simulink model "model_rlseLQR"  (R2018b)
settings: Solver=VariableStepAuto  StartTime=0.0  StopTime=2  RelTol=1e-3
values from neighbouring files (symbols this model uses):
  A_long = [-0.127582199485 -0.120326518027 0.0123230287539 1.06961513757 -0.67567396364 -4.05064303254 -0.0530588085475 -1.81350154459 -15.9023430516 -51.0981546265 -0.573740058259 -35.7720899763 ... (16 elements, 4x4)]    [env_vars.mat]
  B_long = [3.87534978111  10.1410705056; 5.16747566432  -0.750644051383; -0.972922039439  0.0330465441648; -66.5738506051  0.29117538195]    [env_vars.mat]
  euler_0 = deg2rad([5,5,0])    [Linearize.m]    (also in env_vars.mat = [0.0872664625997 0.0872664625997 0])
  K_lat = [4.17654229775  1.2715659909  0.259712133105; 6.03556648418  1.7716700746  0.955044544874]    [env_vars.mat]
  K_long = lqr(A,B,Q,R,N)    [KlongRLSE.m]    (also in env_vars.mat = [-0.0131288079248  0.201593133818  -1.33138461086  -0.241030)
  Klqr = [-0.0154609901399  0.183342172824  -1.54713654668  -0.245681114058; 0.0136126900225  -0.0100908215941  0.035031817911  0.00688258529699]    [env_vars.mat]
  omega_0 = [0,0,0]    [Linearize.m]    (also in env_vars.mat = [0 0 0])
  P = M^(-1)    [LSE.m]    (also in RLSE.m = P*(I - XU*XU'*P/(alpha+XU'*P*XU)); RLSESIM.m = eye(6)*100; RLSE_ff.m = alpha^2*P*(I - XU*XU'*P/(R/alpha^2+XU'*P*XU)); RLSE_klm.m = (I-K*XU')*P)
  phi_cmd = 0    [Linearize.m]    (also in env_vars.mat)
  r = false    [KlongRLSE.m]
  TAS_cmd = 12    [Linearize.m]    (also in env_vars.mat)
  theta_cmd = 0    [Linearize.m]    (also in env_vars.mat)
  TRIM =     [env_vars.mat]
  u_trim_long = u_trim([2 4])    [Linearize.m]    (also in env_vars.mat = [0.0367583336466 0.362566575663])
  UAV =     [env_vars.mat]    (also in loadDATCOMmodel.m = raw{1,1})
  Vb_0 = [13    1   -0.15]    [Linearize.m]    (also in Trim_UAV.m = [11 0.5 0.5]; env_vars.mat = [13 1 -0.15])
  w_cmd = 0    [Linearize.m]    (also in env_vars.mat)
  x_trim_long = [TAS_cmd w_cmd 0 0]    [Linearize.m]    (also in env_vars.mat = [12 0 0 0])
undefined symbols (not defined in the file or in its folder): F, MIL, Severe
libraries: aerolibasang x8, aerolibwind2 x3, aerolibadyn x2, aerolibactuator x1, aerolibatmos2 x1, shared6dof x1
settings Model: SimulationMode=accelerator  Creator=Carlos  LastModifiedBy=Carlos
settings OptimizationCC: EfficientMapNaN2IntZero=off
settings HardwareCC: TargetBitPerLong=64  TargetBitPerPointer=64  TargetBitPerSizeT=64  TargetBitPerPtrDiffT=64  TargetLongLongMode=on  TargetIntDivRoundTo=Zero  TargetEndianess=LittleEndian  TargetWordSize=64  TargetHWDeviceType=MATLAB Host  ProdEqTarget=off
settings CodeAppCC: MaxIdLength=128
settings GRTTargetCC: TargetLangStandard=C89/C90 (ANSI)  CombineOutputUpdateFcns=off  GRTInterface=on

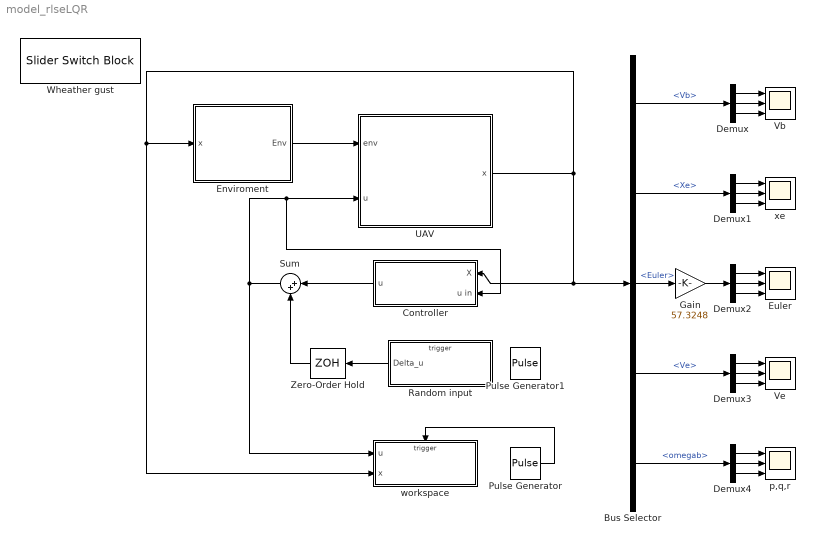
== system model_rlseLQR ==
  Bus Selector : BusSelector  OutputSignals=Vb,Xe,Euler,Ve,omegab
  Controller : Subsystem
  Demux{,1..4} (5 alike) : Demux  Outputs=3
  Enviroment : Subsystem
      mask Display: image('/Volumes/MacintoshHD/Carlos/Downloads/img_7234.png');
  Euler : Scope  NumInputPorts=3
  Gain : Gain  Gain=57.3248
  Pulse Generator : DiscretePulseGenerator  PulseType=Time based  Period=0.02  PulseWidth=5
  Pulse Generator1 : DiscretePulseGenerator  PulseType=Time based  Period=1  PulseWidth=5
  Random input : Subsystem
  Sum : Sum  Inputs=|++
  UAV : Subsystem
      mask Display: image('/Volumes/MacintoshHD/Carlos/Downloads/airplane.gif');
  Vb : Scope  NumInputPorts=3
  Ve : Scope  NumInputPorts=3
  Wheather gust : SliderSwitchBlock  WebBlockId=607
      settings: Values={{'Off', 'On'}, [0 1]}
  Zero-Order Hold : ZeroOrderHold  SampleTime=-1
  p,q,r : Scope  NumInputPorts=3
  workspace : Subsystem  TreatAsAtomicUnit=on
  xe : Scope  NumInputPorts=3
  wires:
  UAV/1("x ") -> Bus Selector/1, Controller/1(X), workspace/2(x), Enviroment/1("x ")
  Enviroment/1(Env) -> UAV/1("env ")
  Demux/1 -> Vb/1
  Bus Selector/1 -> Demux/1  "<Vb>"
  Demux/2 -> Vb/2
  Demux/3 -> Vb/3
  Bus Selector/2 -> Demux1/1  "<Xe>"
  Demux1/1 -> xe/1
  Demux1/2 -> xe/2
  Demux1/3 -> xe/3
  Demux2/1 -> Euler/1
  Demux2/2 -> Euler/2
  Demux2/3 -> Euler/3
  Bus Selector/3 -> Gain/1  "<Euler>"
  Gain/1 -> Demux2/1
  Demux3/3 -> Ve/3
  Bus Selector/4 -> Demux3/1  "<Ve>"
  Demux3/2 -> Ve/2
  Demux3/1 -> Ve/1
  Demux4/1 -> p,q,r/1
  Demux4/3 -> p,q,r/3
  Demux4/2 -> p,q,r/2
  Bus Selector/5 -> Demux4/1  "<omegab>"
  Random input/1(Delta_u) -> Zero-Order Hold/1
  Controller/1(u) -> Sum/1
  Zero-Order Hold/1 -> Sum/2
  Sum/1 -> workspace/1(u), Controller/2(u in), UAV/2(u)
  Pulse Generator/1 -> workspace/Trigger

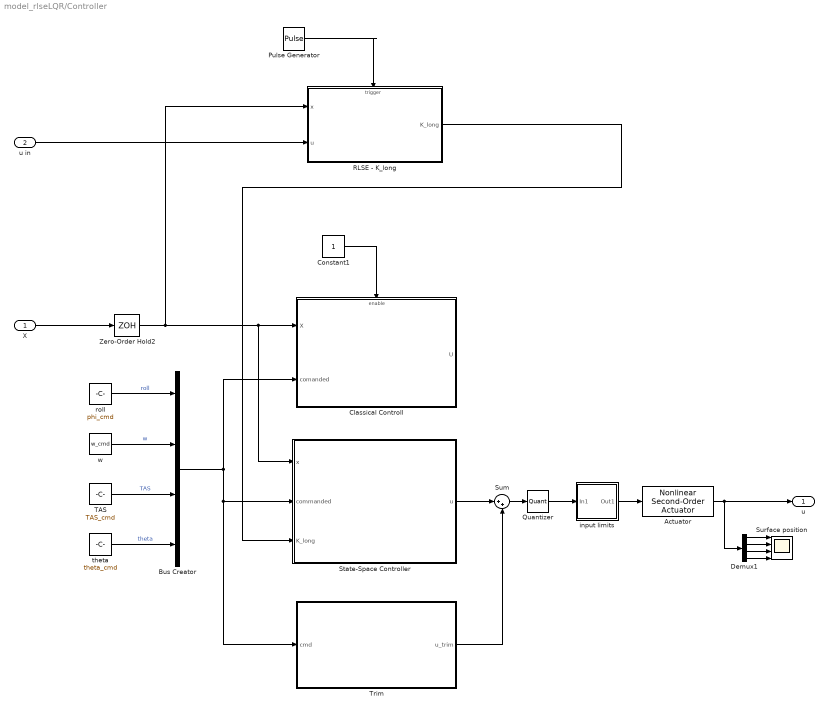
== system model_rlseLQR/Controller ==
  X : Inport
  u in : Inport  Port=2
  Actuator : aerolibactuator/Nonlinear Second-Order Actuator  wn_fin=100  z_fin=0.3  fin_max=1  fin_min=-1  fin_maxrate=2  fin_act_0=0  fin_act_vel=0
      settings: SourceProductName=Aerospace Blockset  SourceProductBaseCode=AE
  Bus Creator : BusCreator  Inputs=4
  Classical Controll : Subsystem  TreatAsAtomicUnit=on
  Constant1 : Constant
  Demux1 : Demux
  Pulse Generator : DiscretePulseGenerator  PulseType=Time based  Period=0.02  PulseWidth=5
  Quantizer : Quantizer  QuantizationInterval=0.004
  RLSE - K_long : Subsystem
  State-Space Controller : Subsystem
  Sum : Sum  Inputs=|++
  Surface position : Scope  NumInputPorts=4
  TAS : Constant  Value=TAS_cmd
  Trim : Subsystem
  Zero-Order Hold2 : ZeroOrderHold  SampleTime=0.01
  input limits : Subsystem
  roll : Constant  Value=phi_cmd
  theta : Constant  Value=theta_cmd
  w : Constant  Value=w_cmd
  u : Outport
  wires:
  Sum/1 -> Quantizer/1
  Constant1/1 -> Classical Controll/Enable
  roll/1 -> Bus Creator/1  "roll"
  Bus Creator/1 -> Classical Controll/2(comanded), Trim/1(cmd), State-Space Controller/2(commanded)
  w/1 -> Bus Creator/2  "w"
  TAS/1 -> Bus Creator/3  "TAS"
  X/1 -> Zero-Order Hold2/1
  Demux1/4 -> Surface position/4
  Demux1/2 -> Surface position/2
  Demux1/1 -> Surface position/1
  Demux1/3 -> Surface position/3
  Zero-Order Hold2/1 -> RLSE - K_long/1(x), State-Space Controller/1(x), Classical Controll/1(X)
  Actuator/1 -> u/1, Demux1/1
  Trim/1(u_trim) -> Sum/2
  theta/1 -> Bus Creator/4  "theta"
  Quantizer/1 -> input limits/1(In1)
  input limits/1(Out1) -> Actuator/1
  Pulse Generator/1 -> RLSE - K_long/Trigger
  RLSE - K_long/1(K_long) -> State-Space Controller/3(K_long)
  u in/1 -> RLSE - K_long/2(u)
  State-Space Controller/1(u) -> Sum/1

== system model_rlseLQR/Enviroment ==
  "x " : Inport
  Bus Creator : BusCreator  Inputs=5
  Bus Selector : BusSelector  OutputSignals=Lhb,Ve,Xe
  Demux : Demux  Outputs=3
  Dot Product : DotProduct  OutDataTypeStr=Inherit: Inherit via internal rule
  ISA Atmosphere Model : aerolibatmos2/ISA Atmosphere Model  custom=off  g=9.80665  gamma=1.4  R=287.0531  L=0.0065  h_trop=11000  h_strat=20000  rho0=1.225  P0=101325  T0=288.15  h0=0
      settings: SourceProductName=Aerospace Blockset
  Scope : Scope  NumInputPorts=3
  Selector : Selector  InputPortWidth=3  IndexOptions=Index vector (dialog)  Indices=[3]  OutputSizes=1
  Wind models : Subsystem
      mask Display: image('/Volumes/MacintoshHD/Carlos/Downloads/f2933471e549912c91ba01f65f304a7c.jpg');
  vt : Sqrt  SaturateOnIntegerOverflow=on
  Env : Outport
  wires:
  Bus Creator/1 -> Env/1
  "x "/1 -> Bus Selector/1
  Bus Selector/3 -> Selector/1  "<Xe>"
  Selector/1 -> ISA Atmosphere Model/1, Wind models/3(altitude)
  ISA Atmosphere Model/4 -> Bus Creator/5  "rho"
  ISA Atmosphere Model/3 -> Bus Creator/4  "P"
  ISA Atmosphere Model/2 -> Bus Creator/3  "a"
  ISA Atmosphere Model/1 -> Bus Creator/2  "T"
  Wind models/1(ug,vg,wg) -> Bus Creator/1, Demux/1  "ug"
  Bus Selector/1 -> Wind models/1(Lhb)  "<Lhb>"
  Dot Product/1 -> vt/1
  Bus Selector/2 -> Dot Product/1, Dot Product/2  "<Ve>"
  vt/1 -> Wind models/2(Airspeed)  "v"
  Demux/1 -> Scope/1
  Demux/2 -> Scope/2
  Demux/3 -> Scope/3

== system model_rlseLQR/Random input ==
  Trigger : TriggerPort  VariantControl=Variant  PortDimensions=1
  random imput vector : MATLAB Function  TreatAsAtomicUnit=on
  Delta_u : Outport
  wires:
  random imput vector/1(y) -> Delta_u/1

== system model_rlseLQR/UAV ==
  "env " : Inport
  u : Inport  Port=2
  6DOF (Euler Angles) : shared6dof/6DOF (Euler Angles)  units=Metric (MKS)  mtype=Fixed  rep=Euler Angles  xme_0=X_0  Vm_0=Vb_0  eul_0=euler_0  pm_0=omega_0  mass_0=UAV.mass  mass_e=0.5  mass_f=2.0  inertia=UAV.Icg  inertia_e=eye(3)  inertia_f=2*eye(3)  k_quat=1.0  vre_flag=on  abi_flag=on  aMode=0  xme_statename=''  Vm_statename=''  eul_statename=''  quat_statename=''  pm_statename=''  mass_statename=''
      settings: SourceProductBaseCode=AE
  Add : Sum  Inputs=3
  "Aero " : Subsystem
  Bus Creator : BusCreator  Inputs=9
  Gravity : Subsystem
  Moto/Propulsion : Subsystem
  Selector : Selector  InputPortWidth=4  IndexOptions=Index vector (dialog)  Indices=[4]  OutputSizes=1
  Sum1 : Sum  Inputs=|++
  "x " : Outport
  wires:
  "env "/1 -> "Aero "/2("Env ")
  6DOF (Euler Angles)/1 -> Bus Creator/1  "Ve"
  6DOF (Euler Angles)/2 -> Bus Creator/2  "Xe"
  6DOF (Euler Angles)/3 -> Bus Creator/3  "Euler"
  6DOF (Euler Angles)/4 -> Bus Creator/4  "Lhb"
  6DOF (Euler Angles)/5 -> [Vb], Bus Creator/5  "Vb"
  Bus Creator/1 -> "Aero "/1("X "), Gravity/1(X), "x "/1
  6DOF (Euler Angles)/6 -> Bus Creator/6  "omegab"
  "Aero "/2("M ") -> Sum1/1
  Moto/Propulsion/2(M) -> Sum1/2
  Selector/1 -> Moto/Propulsion/1(deltap)
  Add/1 -> 6DOF (Euler Angles)/1
  "Aero "/1(F) -> Add/2
  Moto/Propulsion/1(F) -> Add/3
  Sum1/1 -> 6DOF (Euler Angles)/2
  Gravity/1(Fg) -> Add/1
  6DOF (Euler Angles)/7 -> Bus Creator/7  "domegab"
  6DOF (Euler Angles)/8 -> Bus Creator/8  "Abb"
  6DOF (Euler Angles)/9 -> Bus Creator/9  "Abe"
  u/1 -> "Aero "/3(u), Selector/1
  [Vb] -> Moto/Propulsion/2(Vb)

== system model_rlseLQR/workspace ==
  u : Inport
  x : Inport  Port=2
  Trigger : TriggerPort  VariantControl=Variant
  Bus Selector : BusSelector  OutputSignals=Vb,Ve,Euler,omegab,Euler,omegab
  Demux : Demux  Outputs=2
  "Incidence, Sideslip, & Airspeed" : aerolibasang/Incidence, Sideslip, & Airspeed
      settings: SourceProductName=Aerospace Blockset
  Mux : Mux
  Mux1 : Mux
  Selector : Selector  InputPortWidth=4  IndexOptions=Index vector (dialog)  Indices=[2 4]  OutputSizes=1
  Selector1 : Selector  InputPortWidth=4  IndexOptions=Index vector (dialog)  Indices=[1 3]  OutputSizes=1
  Terminator : Terminator
  To Workspace : ToWorkspace  VariableName=u_long  SaveFormat=Timeseries  SampleTime=-1
  To Workspace1 : ToWorkspace  VariableName=x_long  SaveFormat=Timeseries  SampleTime=-1
  To Workspace2 : ToWorkspace  VariableName=u_lat  SaveFormat=Timeseries  SampleTime=-1
  To Workspace3 : ToWorkspace  VariableName=x_lat  SaveFormat=Timeseries  SampleTime=-1
  p,r : Selector  InputPortWidth=3  IndexOptions=Index vector (dialog)  Indices=[1 3]  OutputSizes=1
  phi : Selector  InputPortWidth=3  IndexOptions=Index vector (dialog)  Indices=[1]  OutputSizes=1
  q : Selector  InputPortWidth=3  IndexOptions=Index vector (dialog)  Indices=[2]  OutputSizes=1
  theta : Selector  InputPortWidth=3  IndexOptions=Index vector (dialog)  Indices=[2]  OutputSizes=1
  w : Selector  InputPortWidth=3  IndexOptions=Index vector (dialog)  Indices=[3]  OutputSizes=1
  wires:
  x/1 -> Bus Selector/1
  Bus Selector/2 -> w/1  "<Ve>"
  Bus Selector/3 -> theta/1  "<Euler>"
  Bus Selector/4 -> q/1  "<omegab>"
  Selector/1 -> To Workspace/1
  Mux/1 -> To Workspace1/1
  q/1 -> Mux/4
  theta/1 -> Mux/3
  w/1 -> Mux/2
  Bus Selector/1 -> "Incidence, Sideslip, & Airspeed"/1  "<Vb>"
  "Incidence, Sideslip, & Airspeed"/1 -> Terminator/1
  "Incidence, Sideslip, & Airspeed"/2 -> Mux1/2
  "Incidence, Sideslip, & Airspeed"/3 -> Mux/1
  Selector1/1 -> To Workspace2/1
  u/1 -> Selector1/1, Selector/1
  Bus Selector/6 -> p,r/1  "<omegab>"
  Bus Selector/5 -> phi/1  "<Euler>"
  p,r/1 -> Demux/1
  phi/1 -> Mux1/1
  Demux/2 -> Mux1/4
  Demux/1 -> Mux1/3
  Mux1/1 -> To Workspace3/1

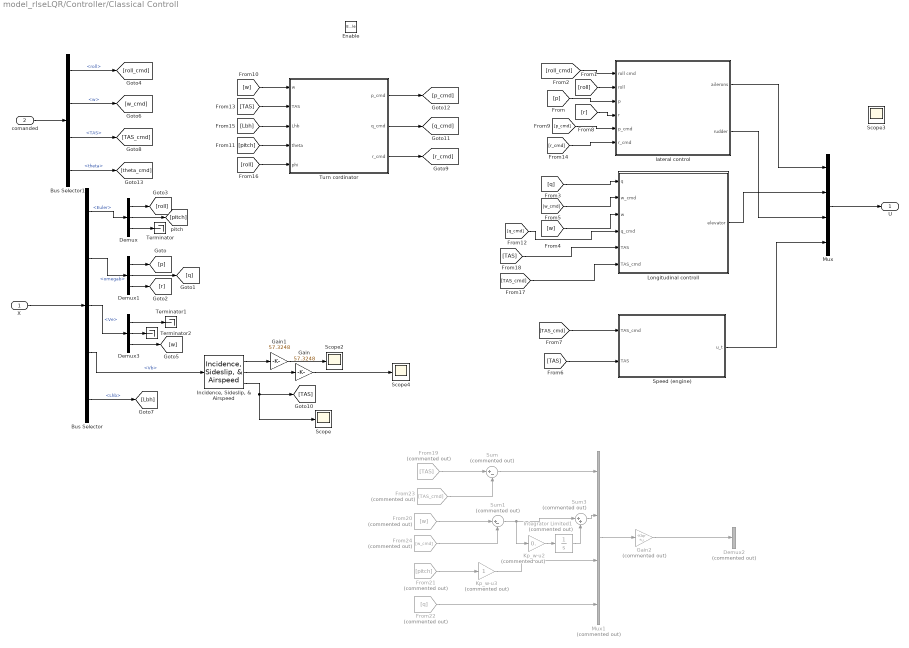
== system model_rlseLQR/Controller/Classical Controll ==
  X : Inport
  comanded : Inport  Port=2
  Enable : EnablePort
  Bus Selector : BusSelector  OutputSignals=Euler,omegab,Ve,Vb,Lhb
  Bus Selector1 : BusSelector  OutputSignals=roll,w,TAS,theta
  Demux : Demux  Outputs=3
  Demux1 : Demux  Outputs=3
  Demux2 : Demux  Commented=on  Outputs=2
  Demux3 : Demux  Outputs=3
  From19 : From  Commented=on  GotoTag=TAS
  From20 : From  Commented=on  GotoTag=w
  From21 : From  Commented=on  GotoTag=pitch
  From22 : From  Commented=on  GotoTag=q
  From23 : From  Commented=on  GotoTag=TAS_cmd
  From24 : From  Commented=on  GotoTag=w_cmd
  Gain : Gain  Gain=57.3248
  Gain1 : Gain  Gain=57.3248
  Gain2 : Gain  Commented=on  Gain=-Klqr  Multiplication=Matrix(K*u)
  "Incidence, Sideslip, & Airspeed" : aerolibasang/Incidence, Sideslip, & Airspeed
      settings: SourceProductName=Aerospace Blockset
  Integrator Limited1 : Integrator  Commented=on  LimitOutput=on  UpperSaturationLimit=2  LowerSaturationLimit=-2
  Kp_w-u2 : Gain  Commented=on  Gain=0.
  Kp_w-u3 : Gain  Commented=on
  Longitudinal controll : Subsystem
  Mux : Mux
  Mux1 : Mux  Commented=on
  Scope{,2..4} (4 alike) : Scope
  Speed (engine) : Subsystem
  Sum : Sum  Commented=on  Inputs=|+-
  Sum1 : Sum  Commented=on  Inputs=|+-
  Sum3 : Sum  Commented=on  Inputs=|++
  Terminator : Terminator
  Terminator1 : Terminator
  Terminator2 : Terminator
  Turn cordinator : Subsystem
  lateral control : Subsystem
  U : Outport
  wires:
  X/1 -> Bus Selector/1
  Bus Selector/1 -> Demux/1  "<Euler>"
  Bus Selector/2 -> Demux1/1  "<omegab>"
  Bus Selector/3 -> Demux3/1  "<Ve>"
  Demux1/1 -> [p]
  Demux1/2 -> [q]
  Demux1/3 -> [r]
  Mux/1 -> U/1
  Demux/1 -> [roll]
  comanded/1 -> Bus Selector1/1
  Bus Selector1/1 -> [roll_cmd]  "<roll>"
  Demux3/3 -> [w]
  Bus Selector1/2 -> [w_cmd]  "<w>"
  [roll_cmd] -> lateral control/1(roll cmd)
  [roll] -> lateral control/2(roll)
  [p] -> lateral control/3(p)
  lateral control/1(ailerons) -> Mux/1
  Bus Selector/4 -> "Incidence, Sideslip, & Airspeed"/1  "<Vb>"
  Bus Selector1/3 -> [TAS_cmd]  "<TAS>"
  "Incidence, Sideslip, & Airspeed"/1 -> Gain1/1
  "Incidence, Sideslip, & Airspeed"/2 -> Gain/1
  Gain/1 -> Scope4/1
  [q] -> Longitudinal controll/1(q)
  [w_cmd] -> Longitudinal controll/2(w_cmd)
  [w] -> Longitudinal controll/3(w)
  lateral control/2(rudder) -> Mux/3
  [r] -> lateral control/4(r)
  [p_cmd] -> lateral control/5(p_cmd)
  [TAS_cmd] -> Speed (engine)/1(TAS_cmd)
  [TAS] -> Speed (engine)/2(TAS)
  [q_cmd] -> Longitudinal controll/4(q_cmd)
  Gain1/1 -> Scope2/1
  Demux/2 -> [pitch]
  [r_cmd] -> lateral control/6(r_cmd)
  "Incidence, Sideslip, & Airspeed"/3 -> [TAS], Scope/1
  Demux/3 -> Terminator/1
  Demux3/1 -> Terminator1/1
  Demux3/2 -> Terminator2/1
  [TAS] -> Turn cordinator/2(TAS)
  Bus Selector/5 -> [Lbh]  "<Lhb>"
  [Lbh] -> Turn cordinator/3(Lhb)
  Turn cordinator/2(q_cmd) -> [q_cmd]
  Turn cordinator/3(r_cmd) -> [r_cmd]
  Turn cordinator/1(p_cmd) -> [p_cmd]
  [w] -> Turn cordinator/1(w)
  [pitch] -> Turn cordinator/4(theta)
  [roll] -> Turn cordinator/5(phi)
  [TAS_cmd] -> Longitudinal controll/6(TAS_cmd)
  [TAS] -> Longitudinal controll/5(TAS)
  From24/1 -> Sum1/2
  From20/1 -> Sum1/1
  From23/1 -> Sum/2
  From19/1 -> Sum/1
  From21/1 -> Kp_w-u3/1
  From22/1 -> Mux1/4
  Mux1/1 -> Gain2/1
  Integrator Limited1/1 -> Sum3/2
  Kp_w-u2/1 -> Integrator Limited1/1
  Sum1/1 -> Kp_w-u2/1, Sum3/1
  Sum3/1 -> Mux1/2
  Kp_w-u3/1 -> Mux1/3
  Sum/1 -> Mux1/1
  Gain2/1 -> Demux2/1
  Speed (engine)/1(u_t) -> Mux/4
  Longitudinal controll/1(elevator) -> Mux/2
  Bus Selector1/4 -> [theta_cmd]  "<theta>"

== system model_rlseLQR/Controller/RLSE - K_long ==
  x : Inport
  u : Inport  Port=2
  Trigger : TriggerPort  VariantControl=Variant  PortDimensions=1
  Bus Selector : BusSelector  OutputSignals=Vb,Ve,Euler,omegab
  Gain : Gain  Gain=50
  "Incidence, Sideslip, & Airspeed" : aerolibasang/Incidence, Sideslip, & Airspeed
      settings: SourceProductName=Aerospace Blockset
  Memory : Memory  InitialCondition=u_trim_long  InheritSampleTime=on
  Memory1 : Memory  InitialCondition=[Vb_0(1) 0 euler_0(2) omega_0(2)]  InheritSampleTime=on
  Mux : Mux
  RLSE & LQR : Subsystem
  Selector : Selector  InputPortWidth=4  IndexOptions=Index vector (dialog)  Indices=[2 4]  OutputSizes=1
  Subtract : Sum  Inputs=-+
  Terminator : Terminator
  Terminator1 : Terminator
  q : Selector  InputPortWidth=3  IndexOptions=Index vector (dialog)  Indices=[2]  OutputSizes=1
  theta : Selector  InputPortWidth=3  IndexOptions=Index vector (dialog)  Indices=[2]  OutputSizes=1
  w : Selector  InputPortWidth=3  IndexOptions=Index vector (dialog)  Indices=[3]  OutputSizes=1
  K_long : Outport
  wires:
  u/1 -> Selector/1
  Subtract/1 -> Gain/1  "∆x"
  Gain/1 -> RLSE & LQR/2(dx)  "dx"
  x/1 -> Bus Selector/1
  w/1 -> Mux/2
  theta/1 -> Mux/3
  q/1 -> Mux/4
  Bus Selector/1 -> "Incidence, Sideslip, & Airspeed"/1  "<Vb>"
  Bus Selector/2 -> w/1  "<Ve>"
  Bus Selector/3 -> theta/1  "<Euler>"
  Bus Selector/4 -> q/1  "<omegab>"
  "Incidence, Sideslip, & Airspeed"/3 -> Mux/1
  "Incidence, Sideslip, & Airspeed"/2 -> Terminator/1
  "Incidence, Sideslip, & Airspeed"/1 -> Terminator1/1
  Memory1/1 -> RLSE & LQR/1(x), Subtract/1
  Selector/1 -> Memory/1
  Mux/1 -> Subtract/2, Memory1/1
  RLSE & LQR/1(K_long) -> K_long/1
  Memory/1 -> RLSE & LQR/3(u)

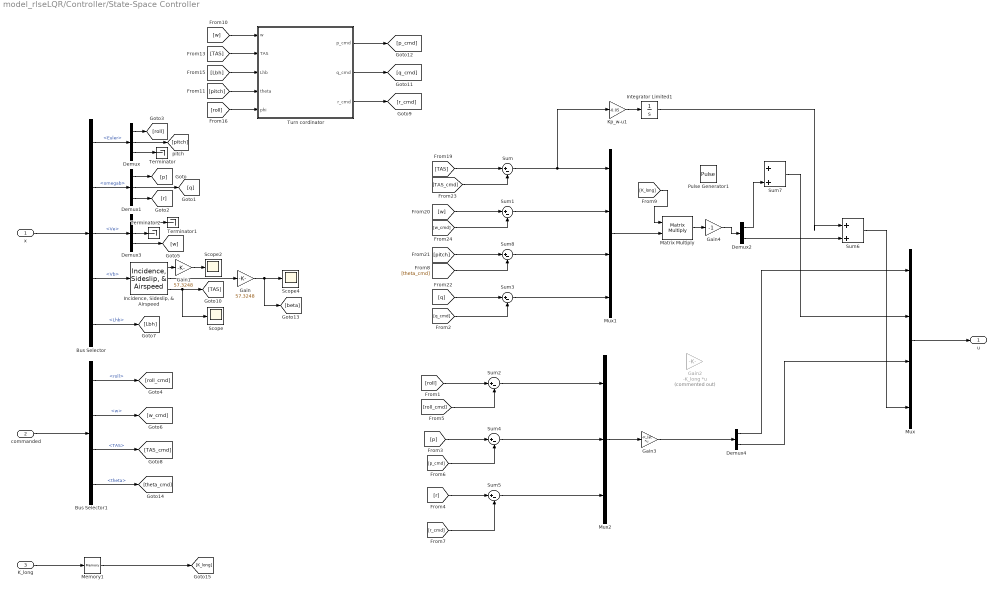
== system model_rlseLQR/Controller/State-Space Controller ==
  x : Inport
  commanded : Inport  Port=2
  K_long : Inport  Port=3
  Bus Selector : BusSelector  OutputSignals=Euler,omegab,Ve,Vb,Lhb
  Bus Selector1 : BusSelector  OutputSignals=roll,w,TAS,theta
  Demux : Demux  Outputs=3
  Demux1 : Demux  Outputs=3
  Demux2 : Demux  Outputs=2
  Demux3 : Demux  Outputs=3
  Demux4 : Demux  Outputs=2
  Gain : Gain  Gain=57.3248
  Gain1 : Gain  Gain=57.3248
  Gain2 : Gain  Commented=on  Gain=-K_long  Multiplication=Matrix(K*u)
  Gain3 : Gain  Gain=-K_lat  Multiplication=Matrix(K*u)
  Gain4 : Gain  Gain=-1
  "Incidence, Sideslip, & Airspeed" : aerolibasang/Incidence, Sideslip, & Airspeed
      settings: SourceProductName=Aerospace Blockset
  Integrator Limited1 : Integrator  LimitOutput=on  UpperSaturationLimit=0.3  LowerSaturationLimit=-0.3
  Kp_w-u1 : Gain  Gain=-0.05
  Matrix Multiply : Product  Multiplication=Matrix(*)
  Memory1 : Memory  InitialCondition=K_long  InheritSampleTime=on
  Mux : Mux
  Mux1 : Mux
  Mux2 : Mux  Inputs=3
  Pulse Generator1 : DiscretePulseGenerator  PulseType=Time based  Amplitude=0.1  Period=1  PulseWidth=10
  Scope : Scope
  Scope2 : Scope
  Scope4 : Scope
  Sum{,1..5,8} (7 alike) : Sum  Inputs=|+-
  Sum6 : Sum  Inputs=|++
  Sum7 : Sum  Inputs=|++
  Terminator : Terminator
  Terminator1 : Terminator
  Terminator2 : Terminator
  Turn cordinator : Subsystem
  u : Outport
  wires:
  Bus Selector1/1 -> [roll_cmd]  "<roll>"
  Bus Selector1/2 -> [w_cmd]  "<w>"
  Bus Selector1/3 -> [TAS_cmd]  "<TAS>"
  commanded/1 -> Bus Selector1/1
  [w_cmd] -> Sum1/2
  [TAS_cmd] -> Sum/2
  [w] -> Sum1/1
  [TAS] -> Sum/1
  Turn cordinator/2(q_cmd) -> [q_cmd]
  Turn cordinator/3(r_cmd) -> [r_cmd]
  Turn cordinator/1(p_cmd) -> [p_cmd]
  [w] -> Turn cordinator/1(w)
  [TAS] -> Turn cordinator/2(TAS)
  [pitch] -> Turn cordinator/4(theta)
  [roll] -> Turn cordinator/5(phi)
  [Lbh] -> Turn cordinator/3(Lhb)
  Bus Selector/1 -> Demux/1  "<Euler>"
  Demux/1 -> [roll]
  Demux3/3 -> [w]
  Bus Selector/3 -> Demux3/1  "<Ve>"
  Bus Selector/2 -> Demux1/1  "<omegab>"
  Gain/1 -> Scope4/1, [beta]
  Demux1/3 -> [r]
  Demux3/1 -> Terminator1/1
  Demux1/1 -> [p]
  Bus Selector/5 -> [Lbh]  "<Lhb>"
  Demux/3 -> Terminator/1
  "Incidence, Sideslip, & Airspeed"/3 -> [TAS], Scope/1
  Demux1/2 -> [q]
  "Incidence, Sideslip, & Airspeed"/2 -> Gain/1
  Demux3/2 -> Terminator2/1
  "Incidence, Sideslip, & Airspeed"/1 -> Gain1/1
  Gain1/1 -> Scope2/1
  Bus Selector/4 -> "Incidence, Sideslip, & Airspeed"/1  "<Vb>"
  Demux/2 -> [pitch]
  x/1 -> Bus Selector/1
  Mux2/1 -> Gain3/1
  Gain3/1 -> Demux4/1
  [roll_cmd] -> Sum2/2
  [roll] -> Sum2/1
  Mux/1 -> u/1
  Demux4/1 -> Mux/1
  Demux4/2 -> Mux/3
  Sum2/1 -> Mux2/1
  Sum1/1 -> Mux1/2
  [q] -> Sum3/1
  Sum3/1 -> Mux1/4
  [q_cmd] -> Sum3/2
  [p] -> Sum4/1
  Sum4/1 -> Mux2/2
  [p_cmd] -> Sum4/2
  [r] -> Sum5/1
  Sum5/1 -> Mux2/3
  [r_cmd] -> Sum5/2
  Integrator Limited1/1 -> Sum6/1
  Kp_w-u1/1 -> Integrator Limited1/1
  Sum/1 -> Kp_w-u1/1, Mux1/1
  Demux2/2 -> Sum6/2
  Sum6/1 -> Mux/4
  Demux2/1 -> Sum7/2
  Sum7/1 -> Mux/2
  Bus Selector1/4 -> [theta_cmd]  "<theta>"
  [theta_cmd] -> Sum8/2
  [pitch] -> Sum8/1
  Sum8/1 -> Mux1/3
  K_long/1 -> Memory1/1
  [K_long] -> Matrix Multiply/1
  Memory1/1 -> [K_long]
  Matrix Multiply/1 -> Gain4/1
  Mux1/1 -> Matrix Multiply/2
  Gain4/1 -> Demux2/1

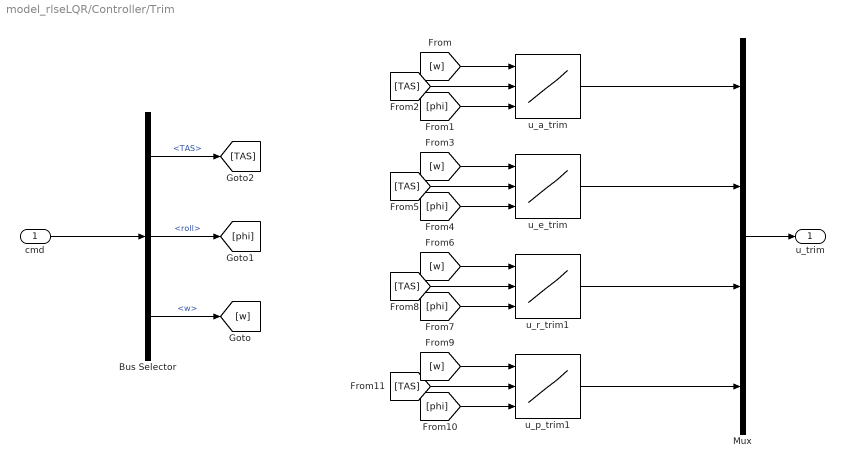
== system model_rlseLQR/Controller/Trim ==
  cmd : Inport
  Bus Selector : BusSelector  OutputSignals=TAS,roll,w
  Mux : Mux
  u_a_trim : Lookup_n-D  NumberOfTableDimensions=3  BreakpointsForDimension1=TRIM.w  BreakpointsForDimension2=TRIM.TAS  BreakpointsForDimension3=TRIM.phi  Table=TRIM.u_a  InternalRulePriority=Speed  RndMeth=Simplest  InputSameDT=on
  u_e_trim : Lookup_n-D  NumberOfTableDimensions=3  BreakpointsForDimension1=TRIM.w  BreakpointsForDimension2=TRIM.TAS  BreakpointsForDimension3=TRIM.phi  Table=TRIM.u_e  InternalRulePriority=Speed  RndMeth=Simplest  InputSameDT=on
  u_p_trim1 : Lookup_n-D  NumberOfTableDimensions=3  BreakpointsForDimension1=TRIM.w  BreakpointsForDimension2=TRIM.TAS  BreakpointsForDimension3=TRIM.phi  Table=TRIM.u_p  InternalRulePriority=Speed  RndMeth=Simplest  InputSameDT=on
  u_r_trim1 : Lookup_n-D  NumberOfTableDimensions=3  BreakpointsForDimension1=TRIM.w  BreakpointsForDimension2=TRIM.TAS  BreakpointsForDimension3=TRIM.phi  Table=TRIM.u_r  InternalRulePriority=Speed  RndMeth=Simplest  InputSameDT=on
  u_trim : Outport
  wires:
  Mux/1 -> u_trim/1
  u_a_trim/1 -> Mux/1
  cmd/1 -> Bus Selector/1
  [w] -> u_a_trim/1
  [phi] -> u_a_trim/3
  [TAS] -> u_a_trim/2
  [TAS] -> u_e_trim/2
  [w] -> u_e_trim/1
  [phi] -> u_e_trim/3
  u_e_trim/1 -> Mux/2
  u_r_trim1/1 -> Mux/3
  [TAS] -> u_r_trim1/2
  [w] -> u_r_trim1/1
  [phi] -> u_r_trim1/3
  u_p_trim1/1 -> Mux/4
  [TAS] -> u_p_trim1/2
  [w] -> u_p_trim1/1
  [phi] -> u_p_trim1/3
  Bus Selector/1 -> [TAS]  "<TAS>"
  Bus Selector/2 -> [phi]  "<roll>"
  Bus Selector/3 -> [w]  "<w>"

== system model_rlseLQR/Controller/input limits ==
  In1 : Inport
  Demux : Demux
  Mux : Mux
  Saturation : Saturate  UpperLimit=1  LowerLimit=-1
  Saturation1 : Saturate  UpperLimit=1  LowerLimit=-1
  Saturation2 : Saturate  UpperLimit=1  LowerLimit=-1
  Saturation3 : Saturate  UpperLimit=1  LowerLimit=0
  Out1 : Outport
  wires:
  In1/1 -> Demux/1
  Demux/1 -> Saturation/1
  Demux/2 -> Saturation1/1
  Demux/3 -> Saturation2/1
  Demux/4 -> Saturation3/1
  Saturation/1 -> Mux/1
  Mux/1 -> Out1/1
  Saturation3/1 -> Mux/4
  Saturation2/1 -> Mux/3
  Saturation1/1 -> Mux/2

== system model_rlseLQR/Enviroment/Wind models ==
  Lhb : Inport
  Airspeed : Inport  Port=2
  altitude : Inport  Port=3
  Discrete Wind Gust Model : aerolibwind2/Discrete Wind Gust Model  units=Metric (MKS)  Gx=off  Gy=off  Gz=off  t_0=20  d_m=[10 10 10]  v_m=[1 1 1]
      settings: SourceProductName=Aerospace Blockset
  Dryden Wind Turbulence Model (Continuous (+q +r)) : aerolibwind2/Dryden Wind Turbulence Model  (Continuous (+q -r))  units=Metric (MKS)  spec=MIL-F-8785C  model=Discrete Dryden (+q +r)  W20=2  Wdeg=90  TurbProb=10^-5 - Severe  L_high=533.4  Wingspan=2  ts=0.1  Seed=[23341 23342 23343 23344]  T_on=on
      settings: SourceProductName=Aerospace Blockset
  Scope : Scope
  Sum : Sum  Inputs=+++  SaturateOnIntegerOverflow=on  InputSameDT=on  OutDataTypeStr=Inherit: Same as first input
  Terminator : Terminator
  Wind Shear Model : aerolibwind2/Wind Shear Model  units=Metric (MKS)  phase=Category C - Terminal Flight Phase  W_20=5  Wdeg=90
      settings: SourceProductName=Aerospace Blockset
  ug,vg,wg : Outport  Unit=m/s
  wires:
  Discrete Wind Gust Model/1 -> Sum/3
  altitude/1 -> Wind Shear Model/1, Dryden Wind Turbulence Model (Continuous (+q +r))/1
  Lhb/1 -> Wind Shear Model/2, Dryden Wind Turbulence Model (Continuous (+q +r))/3
  Dryden Wind Turbulence Model (Continuous (+q +r))/2 -> Terminator/1  "WindAngularRates"
  Airspeed/1 -> Dryden Wind Turbulence Model (Continuous (+q +r))/2, Discrete Wind Gust Model/1
  Sum/1 -> Scope/1, ug,vg,wg/1  "WindVelocity"
  Dryden Wind Turbulence Model (Continuous (+q +r))/1 -> Sum/2
  Wind Shear Model/1 -> Sum/1

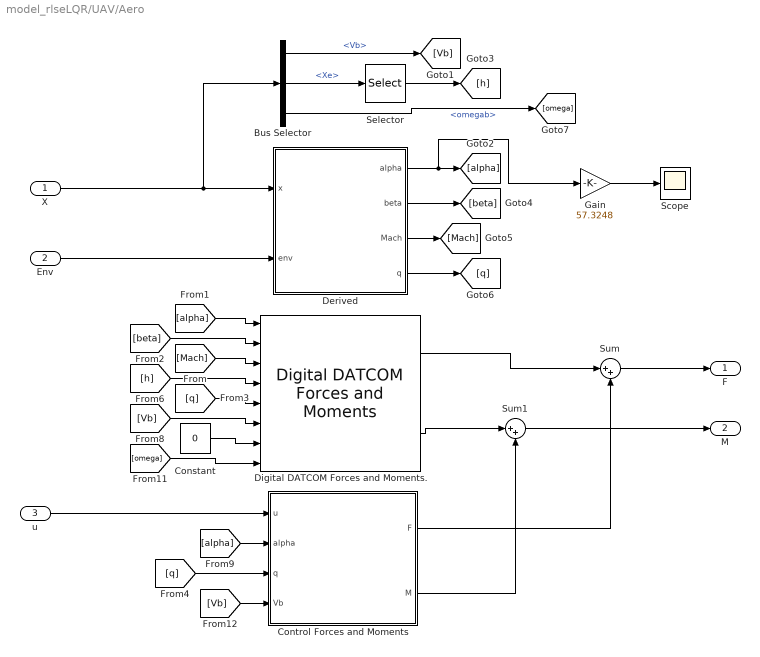
== system model_rlseLQR/UAV/Aero  ==
  "X " : Inport
  "Env " : Inport  Port=2
  u : Inport  Port=3
  Bus Selector : BusSelector  OutputSignals=Vb,Xe,omegab
  Constant : Constant  Value=0
  Control Forces and Moments : Subsystem
  Derived : Subsystem
  Digital DATCOM Forces and Moments. : aerolibadyn/Digital DATCOM Forces and Moments  units=Metric (MKS)  dcase=UAV  fmode=Body  buildno=0  imethod=None - flat  emethod=None - clip  rmethod=Clip to Range  action=None
      settings: SourceProductName=Aerospace Blockset  SourceProductBaseCode=AE
  Gain : Gain  Gain=57.3248
  Scope : Scope
  Selector : Selector  InputPortWidth=3  IndexOptions=Index vector (dialog)  Indices=3  OutputSizes=1
  Sum : Sum  Inputs=|++
  Sum1 : Sum  Inputs=|++
  F : Outport
  "M " : Outport  Port=2
  wires:
  "X "/1 -> Bus Selector/1, Derived/1(x)
  [Mach] -> Digital DATCOM Forces and Moments./3
  Bus Selector/1 -> [Vb]  "<Vb>"
  Digital DATCOM Forces and Moments./2 -> Sum1/1
  Sum1/1 -> "M "/1
  Digital DATCOM Forces and Moments./1 -> Sum/1
  Sum/1 -> F/1
  [q] -> Digital DATCOM Forces and Moments./5
  Control Forces and Moments/1(F) -> Sum/2
  Control Forces and Moments/2(M) -> Sum1/2
  u/1 -> Control Forces and Moments/1(u)
  [q] -> Control Forces and Moments/3(q)
  "Env "/1 -> Derived/2(env)
  Derived/2(beta) -> [beta]
  Derived/4(q) -> [q]
  [alpha] -> Digital DATCOM Forces and Moments./1
  [beta] -> Digital DATCOM Forces and Moments./2
  [h] -> Digital DATCOM Forces and Moments./4
  [Vb] -> Digital DATCOM Forces and Moments./6
  [alpha] -> Control Forces and Moments/2(alpha)
  Bus Selector/2 -> Selector/1  "<Xe>"
  Selector/1 -> [h]
  Bus Selector/3 -> [omega]  "<omegab>"
  Derived/1(alpha) -> Gain/1, [alpha]
  [omega] -> Digital DATCOM Forces and Moments./8
  Derived/3(Mach) -> [Mach]
  Gain/1 -> Scope/1
  [Vb] -> Control Forces and Moments/4(Vb)
  Constant/1 -> Digital DATCOM Forces and Moments./7

== system model_rlseLQR/UAV/Gravity ==
  X : Inport
  Bus Selector : BusSelector  OutputSignals=Lhb
  Constant2 : Constant  Value=[0 0 UAV.mass]
  Gain : Gain  Gain=9.81
  To body Axes : Product  Multiplication=Matrix(*)  SaturateOnIntegerOverflow=on  InputSameDT=on  OutDataTypeStr=Inherit: Same as first input
  Fg : Outport
  wires:
  Bus Selector/1 -> To body Axes/1  "<Lhb>"
  To body Axes/1 -> Fg/1  "Fg"
  X/1 -> Bus Selector/1
  Constant2/1 -> Gain/1
  Gain/1 -> To body Axes/2

== system model_rlseLQR/UAV/Moto//Propulsion ==
  deltap : Inport
  Vb : Inport  Port=2
  Divide : Product  Inputs=*/*
  Divide1 : Product  Inputs=*/*
  Efficiency : Gain  Gain=UAV.eng_eff
  Engine power : Constant  Value=UAV.power
  "Incidence, Sideslip, & Airspeed" : aerolibasang/Incidence, Sideslip, & Airspeed
      settings: SourceProductName=Aerospace Blockset
  Max rpm : Constant  Value=UAV.rpm_max
  Mux : Mux  Inputs=2
  Mux1 : Mux  Inputs=2
  Terminator : Terminator
  Terminator1 : Terminator
  ThrustX1 : Lookup_n-D  NumberOfTableDimensions=1  LookupTableObject=''  BreakpointsForDimension1=(1/6)*(3+([-3:3]))  IndexSearchMethod=Linear search  BeginIndexSearchUsingPreviousIndexResult=on  Table=(0.5*(1+tanh([-3:3])))  ExtrapMethod=Clip  InputSameDT=on
  Ty,Tz : Constant  Value=[0,0]
  Ty,Tz1 : Constant  Value=[0,0]
  rpm2rads : Gain  Gain=0.104719755119660
  F : Outport
  M : Outport  Port=2
  wires:
  Mux/1 -> F/1
  Ty,Tz/1 -> Mux/2
  Ty,Tz1/1 -> Mux1/2
  Mux1/1 -> M/1
  Vb/1 -> "Incidence, Sideslip, & Airspeed"/1
  "Incidence, Sideslip, & Airspeed"/1 -> Terminator/1
  "Incidence, Sideslip, & Airspeed"/2 -> Terminator1/1
  "Incidence, Sideslip, & Airspeed"/3 -> Divide/2
  Engine power/1 -> Divide1/1, Efficiency/1
  ThrustX1/1 -> Divide/3, Divide1/3
  Divide/1 -> Mux/1
  Efficiency/1 -> Divide/1
  deltap/1 -> ThrustX1/1
  Divide1/1 -> Mux1/1
  Max rpm/1 -> rpm2rads/1
  rpm2rads/1 -> Divide1/2

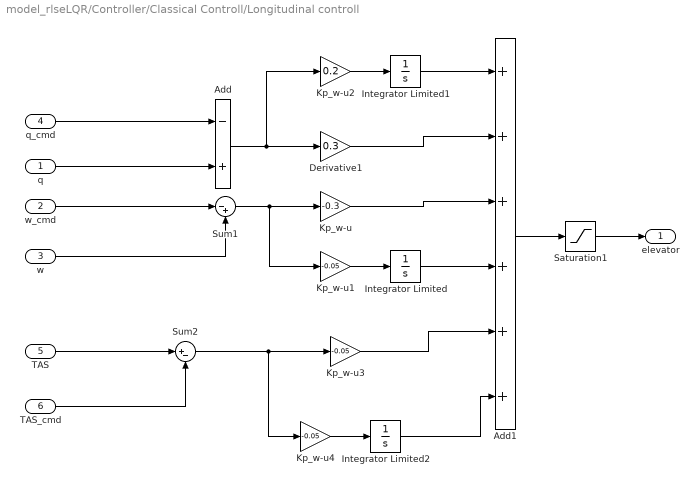
== system model_rlseLQR/Controller/Classical Controll/Longitudinal controll ==
  q : Inport
  w_cmd : Inport  Port=2
  w : Inport  Port=3
  q_cmd : Inport  Port=4
  TAS : Inport  Port=5
  TAS_cmd : Inport  Port=6
  Add : Sum  Inputs=-+
  Add1 : Sum  Inputs=++++++
  Derivative1 : Gain  Gain=0.3
  Integrator Limited : Integrator  LimitOutput=on  UpperSaturationLimit=0.5  LowerSaturationLimit=-0.5
  Integrator Limited1 : Integrator  LimitOutput=on  UpperSaturationLimit=0.25  LowerSaturationLimit=-0.25
  Integrator Limited2 : Integrator  LimitOutput=on  UpperSaturationLimit=0.5  LowerSaturationLimit=-0.5
  Kp_w-u : Gain  Gain=-0.3
  Kp_w-u1 : Gain  Gain=-0.05
  Kp_w-u2 : Gain  Gain=0.2
  Kp_w-u3 : Gain  Gain=-0.05
  Kp_w-u4 : Gain  Gain=-0.05
  Saturation1 : Saturate  UpperLimit=1  LowerLimit=-1
  Sum1 : Sum  Inputs=|-+
  Sum2 : Sum  Inputs=|+-
  elevator : Outport
  wires:
  Saturation1/1 -> elevator/1
  Add1/1 -> Saturation1/1
  w_cmd/1 -> Sum1/1
  Sum1/1 -> Kp_w-u1/1, Kp_w-u/1
  w/1 -> Sum1/2
  Add/1 -> Kp_w-u2/1, Derivative1/1
  q/1 -> Add/2
  Kp_w-u1/1 -> Integrator Limited/1
  q_cmd/1 -> Add/1
  Kp_w-u2/1 -> Integrator Limited1/1
  Integrator Limited/1 -> Add1/4
  Kp_w-u/1 -> Add1/3
  Derivative1/1 -> Add1/2
  Integrator Limited1/1 -> Add1/1
  TAS/1 -> Sum2/1
  TAS_cmd/1 -> Sum2/2
  Kp_w-u3/1 -> Add1/5
  Integrator Limited2/1 -> Add1/6
  Sum2/1 -> Kp_w-u4/1, Kp_w-u3/1
  Kp_w-u4/1 -> Integrator Limited2/1

== system model_rlseLQR/Controller/Classical Controll/Speed (engine) ==
  TAS_cmd : Inport
  TAS : Inport  Port=2
  Add2 : Sum
  Integrator Limited1 : Integrator  LimitOutput=on  UpperSaturationLimit=0.3  LowerSaturationLimit=-0.3
  Kp_w-u1 : Gain  Gain=-0.07
  Saturation2 : Saturate
  Sum2 : Sum  Inputs=|-+
  TAS_prop : Gain  Gain=-0.15
  u_t : Outport
  wires:
  Saturation2/1 -> u_t/1
  TAS_cmd/1 -> Sum2/1
  Add2/1 -> Saturation2/1
  TAS_prop/1 -> Add2/1
  Integrator Limited1/1 -> Add2/2
  TAS/1 -> Sum2/2
  Sum2/1 -> Kp_w-u1/1, TAS_prop/1
  Kp_w-u1/1 -> Integrator Limited1/1

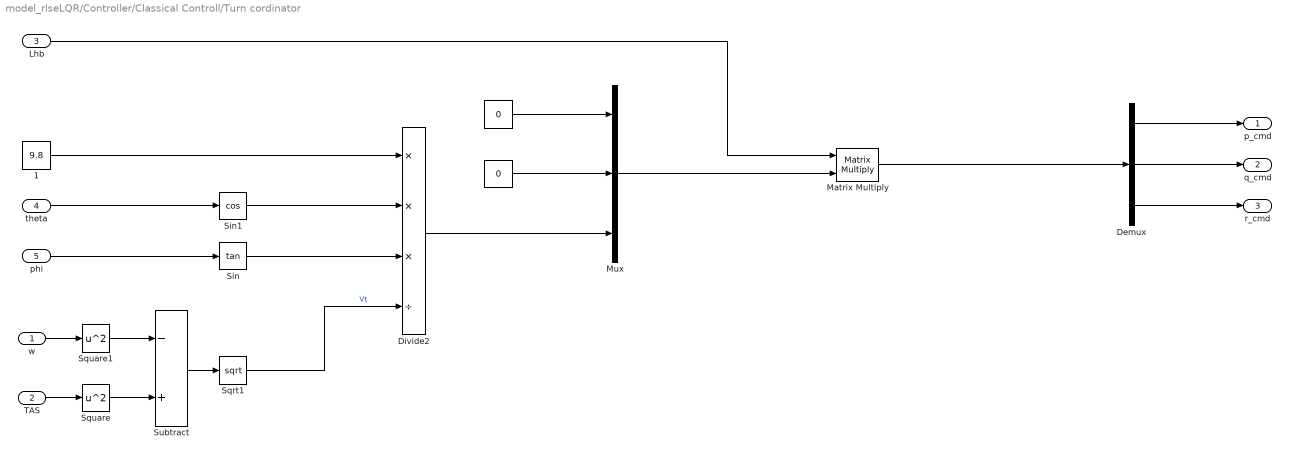
== system model_rlseLQR/Controller/Classical Controll/Turn cordinator ==
  w : Inport
  TAS : Inport  Port=2
  Lhb : Inport  Port=3
  theta : Inport  Port=4
  phi : Inport  Port=5
  " " : Constant  Value=0
  "  " : Constant  Value=0
  " 1" : Constant  Value=9.8
  Demux : Demux  Outputs=3
  Divide2 : Product  Inputs=***/
  Matrix Multiply : Product  Multiplication=Matrix(*)
  Mux : Mux  Inputs=3
  Sin : Trigonometry  Operator=tan  OutputSignalType=real
  Sin1 : Trigonometry  Operator=cos
  Sqrt1 : Sqrt  SaturateOnIntegerOverflow=on
  Square : Math  Operator=square  SaturateOnIntegerOverflow=on
  Square1 : Math  Operator=square  SaturateOnIntegerOverflow=on
  Subtract : Sum  Inputs=-+
  p_cmd : Outport
  q_cmd : Outport  Port=2
  r_cmd : Outport  Port=3
  wires:
  Demux/1 -> p_cmd/1
  Demux/2 -> q_cmd/1
  Demux/3 -> r_cmd/1
  w/1 -> Square1/1
  Square1/1 -> Subtract/1
  Square/1 -> Subtract/2
  Subtract/1 -> Sqrt1/1
  " "/1 -> Mux/1
  theta/1 -> Sin1/1
  phi/1 -> Sin/1
  Sin/1 -> Divide2/3
  Sin1/1 -> Divide2/2
  " 1"/1 -> Divide2/1
  "  "/1 -> Mux/2
  Divide2/1 -> Mux/3
  Lhb/1 -> Matrix Multiply/1
  Mux/1 -> Matrix Multiply/2
  Matrix Multiply/1 -> Demux/1
  TAS/1 -> Square/1
  Sqrt1/1 -> Divide2/4  "Vt"

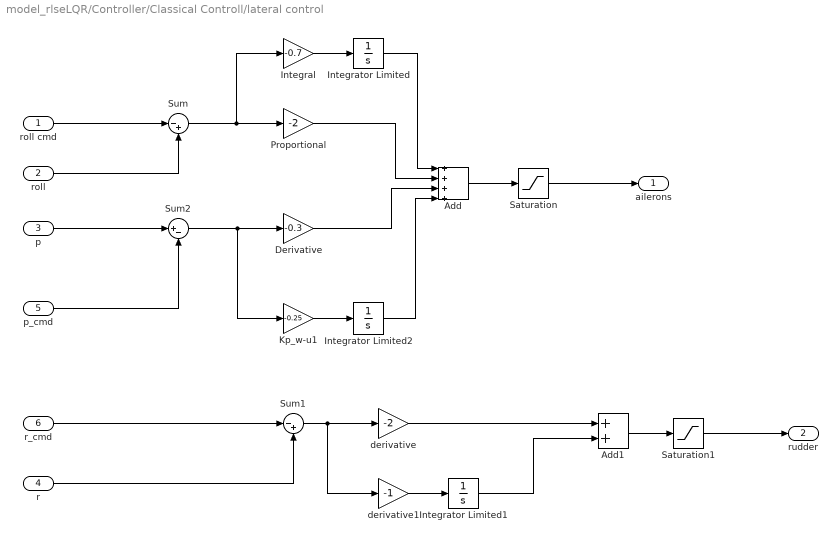
== system model_rlseLQR/Controller/Classical Controll/lateral control ==
  roll cmd : Inport
  roll : Inport  Port=2
  p : Inport  Port=3
  r : Inport  Port=4
  p_cmd : Inport  Port=5
  r_cmd : Inport  Port=6
  Add : Sum  Inputs=++++
  Add1 : Sum
  Derivative : Gain  Gain=-0.3
  Integral : Gain  Gain=-0.7
  Integrator Limited : Integrator  LimitOutput=on  UpperSaturationLimit=0.5  LowerSaturationLimit=-0.5
  Integrator Limited1 : Integrator  LimitOutput=on  UpperSaturationLimit=0.1  LowerSaturationLimit=-0.1
  Integrator Limited2 : Integrator  LimitOutput=on  UpperSaturationLimit=0.25  LowerSaturationLimit=-0.25
  Kp_w-u1 : Gain  Gain=-0.25
  Proportional : Gain  Gain=-2
  Saturation : Saturate  UpperLimit=1  LowerLimit=-1
  Saturation1 : Saturate  UpperLimit=1  LowerLimit=-1
  Sum : Sum  Inputs=|-+
  Sum1 : Sum  Inputs=|-+
  Sum2 : Sum  Inputs=|+-
  derivative : Gain  Gain=-2
  derivative1 : Gain  Gain=-1
  ailerons : Outport
  rudder : Outport  Port=2
  wires:
  roll cmd/1 -> Sum/1
  Saturation/1 -> ailerons/1
  roll/1 -> Sum/2
  Derivative/1 -> Add/3
  Proportional/1 -> Add/2
  Add/1 -> Saturation/1
  Sum/1 -> Proportional/1, Integral/1
  Integral/1 -> Integrator Limited/1
  Integrator Limited/1 -> Add/1
  Add1/1 -> Saturation1/1
  r/1 -> Sum1/2
  Sum1/1 -> derivative1/1, derivative/1
  Integrator Limited1/1 -> Add1/2
  derivative1/1 -> Integrator Limited1/1
  Saturation1/1 -> rudder/1
  r_cmd/1 -> Sum1/1
  p/1 -> Sum2/1
  p_cmd/1 -> Sum2/2
  derivative/1 -> Add1/1
  Sum2/1 -> Kp_w-u1/1, Derivative/1
  Integrator Limited2/1 -> Add/4
  Kp_w-u1/1 -> Integrator Limited2/1

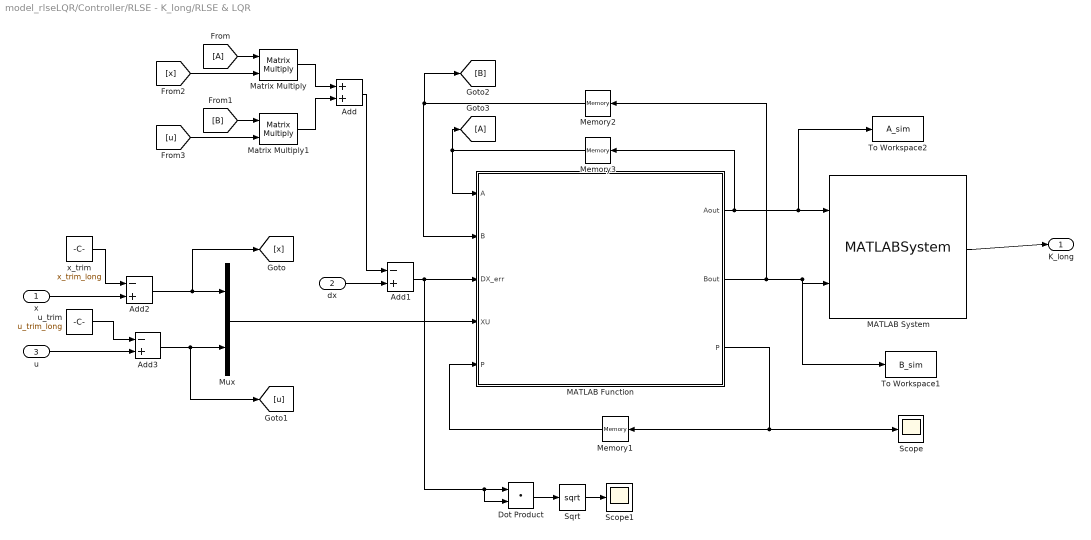
== system model_rlseLQR/Controller/RLSE - K_long/RLSE & LQR ==
  x : Inport
  dx : Inport  Port=2
  u : Inport  Port=3
  Add : Sum
  Add1 : Sum  Inputs=-+
  Add2 : Sum  Inputs=-+
  Add3 : Sum  Inputs=-+
  Dot Product : DotProduct  InputSameDT=on  OutDataTypeStr=Inherit: Inherit via internal rule
  MATLAB Function : MATLAB Function  TreatAsAtomicUnit=on
  MATLAB System : MATLABSystem  System=KlongRLSE  SimulateUsing=Interpreted execution
      mask Type: KlongRLSE
      mask Display:
      | disp('KlongRLSE');
      | port_label('input',1,'A');
      | port_label('input',2,'B');
      | port_label('output',1,'K_long');
  Matrix Multiply : Product  Multiplication=Matrix(*)
  Matrix Multiply1 : Product  Multiplication=Matrix(*)
  Memory1 : Memory  InitialCondition=eye(6)*P  InheritSampleTime=on
  Memory2 : Memory  InitialCondition=B_long  InheritSampleTime=on
  Memory3 : Memory  InitialCondition=A_long  InheritSampleTime=on
  Mux : Mux  Inputs=2
  Scope : Scope
  Scope1 : Scope
  Sqrt : Sqrt  SaturateOnIntegerOverflow=on
  To Workspace1 : ToWorkspace  VariableName=B_sim  SaveFormat=Timeseries  SampleTime=-1
  To Workspace2 : ToWorkspace  VariableName=A_sim  SaveFormat=Timeseries  SampleTime=-1
  u_trim : Constant  Value=u_trim_long
  x_trim : Constant  Value=x_trim_long
  K_long : Outport
  wires:
  Mux/1 -> MATLAB Function/4(XU)
  MATLAB Function/1(Aout) -> Memory3/1, MATLAB System/1, To Workspace2/1
  MATLAB Function/2(Bout) -> Memory2/1, MATLAB System/2, To Workspace1/1
  Memory2/1 -> [B], MATLAB Function/2(B)
  Memory3/1 -> MATLAB Function/1(A), [A]
  Matrix Multiply/1 -> Add/1
  Matrix Multiply1/1 -> Add/2
  [A] -> Matrix Multiply/1
  [B] -> Matrix Multiply1/1
  [u] -> Matrix Multiply1/2
  [x] -> Matrix Multiply/2
  dx/1 -> Add1/2
  Add1/1 -> Dot Product/1, Dot Product/2, MATLAB Function/3(DX_err)
  Add/1 -> Add1/1
  Memory1/1 -> MATLAB Function/5("P ")
  MATLAB Function/3(P) -> Scope/1, Memory1/1
  x/1 -> Add2/2
  Add2/1 -> [x], Mux/1
  u/1 -> Add3/2
  Add3/1 -> [u], Mux/2
  x_trim/1 -> Add2/1
  u_trim/1 -> Add3/1
  MATLAB System/1 -> K_long/1
  Dot Product/1 -> Sqrt/1
  Sqrt/1 -> Scope1/1

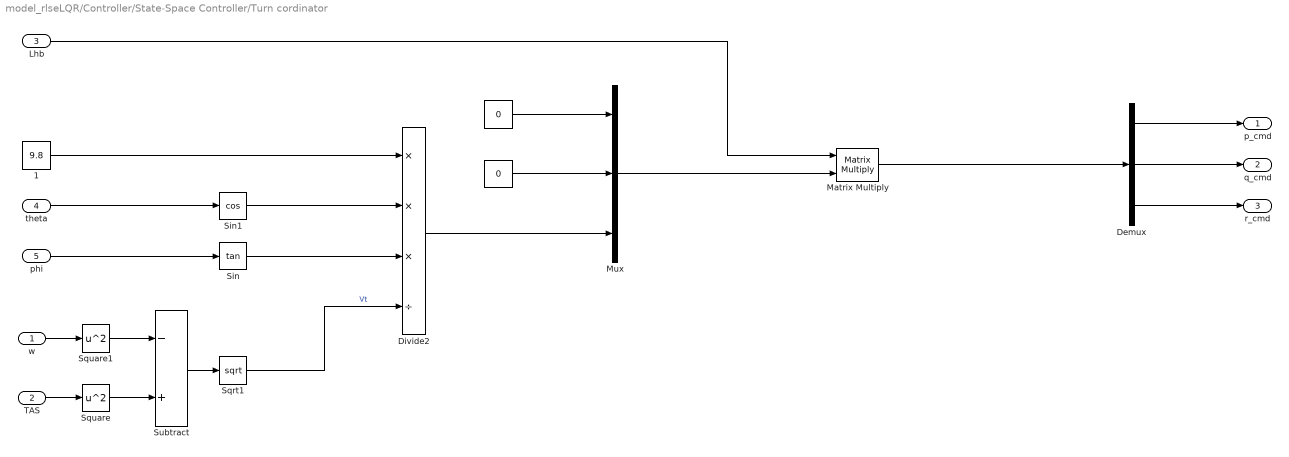
== system model_rlseLQR/Controller/State-Space Controller/Turn cordinator ==
  w : Inport
  TAS : Inport  Port=2
  Lhb : Inport  Port=3
  theta : Inport  Port=4
  phi : Inport  Port=5
  " " : Constant  Value=0
  "  " : Constant  Value=0
  " 1" : Constant  Value=9.8
  Demux : Demux  Outputs=3
  Divide2 : Product  Inputs=***/
  Matrix Multiply : Product  Multiplication=Matrix(*)
  Mux : Mux  Inputs=3
  Sin : Trigonometry  Operator=tan  OutputSignalType=real
  Sin1 : Trigonometry  Operator=cos
  Sqrt1 : Sqrt  SaturateOnIntegerOverflow=on
  Square : Math  Operator=square  SaturateOnIntegerOverflow=on
  Square1 : Math  Operator=square  SaturateOnIntegerOverflow=on
  Subtract : Sum  Inputs=-+
  p_cmd : Outport
  q_cmd : Outport  Port=2
  r_cmd : Outport  Port=3
  wires:
  Demux/1 -> p_cmd/1
  Demux/2 -> q_cmd/1
  Demux/3 -> r_cmd/1
  w/1 -> Square1/1
  Square1/1 -> Subtract/1
  Square/1 -> Subtract/2
  Subtract/1 -> Sqrt1/1
  " "/1 -> Mux/1
  theta/1 -> Sin1/1
  phi/1 -> Sin/1
  Sin/1 -> Divide2/3
  Sin1/1 -> Divide2/2
  " 1"/1 -> Divide2/1
  "  "/1 -> Mux/2
  Divide2/1 -> Mux/3
  Lhb/1 -> Matrix Multiply/1
  Mux/1 -> Matrix Multiply/2
  Matrix Multiply/1 -> Demux/1
  TAS/1 -> Square/1
  Sqrt1/1 -> Divide2/4  "Vt"

== system model_rlseLQR/UAV/Aero /Control Forces and Moments ==
  u : Inport
  alpha : Inport  Port=2
  q : Inport  Port=3
  Vb : Inport  Port=4
  Aero Coefficients : Subsystem
  "Aerodynamic Forces and Moments " : aerolibadyn/Aerodynamic Forces and Moments   inputAxes=Stability  outputForceAxes=Body  outputMomentAxes=Body  S=UAV.sref  b=UAV.blref  cbar=UAV.blref
      settings: SourceProductName=Aerospace Blockset
  F : Outport
  M : Outport  Port=2
  wires:
  "Aerodynamic Forces and Moments "/2 -> M/1
  "Aerodynamic Forces and Moments "/1 -> F/1
  Aero Coefficients/1("Coeff ") -> "Aerodynamic Forces and Moments "/1
  Aero Coefficients/4("Cp ") -> "Aerodynamic Forces and Moments "/4
  alpha/1 -> Aero Coefficients/2(alpha)
  u/1 -> Aero Coefficients/1(u)
  Aero Coefficients/2(qout) -> "Aerodynamic Forces and Moments "/2
  q/1 -> Aero Coefficients/3(q)
  Vb/1 -> "Aerodynamic Forces and Moments "/5
  Aero Coefficients/3("Cg ") -> "Aerodynamic Forces and Moments "/3

== system model_rlseLQR/UAV/Aero /Derived ==
  x : Inport
  env : Inport  Port=2
  Bus Selector : BusSelector  OutputSignals=Vb
  Bus Selector1 : BusSelector  OutputSignals=ug,a,rho
  Dynamic Pressure : aerolibasang/Dynamic Pressure
  Gain : Gain
  "Incidence, Sideslip, & Airspeed" : aerolibasang/Incidence, Sideslip, & Airspeed
      settings: SourceProductName=Aerospace Blockset
  Mach Number : aerolibasang/Mach Number
      settings: SourceProductName=Aerospace Blockset  SourceProductBaseCode=AE
  Sum : Sum  Inputs=|+-
  Terminator : Terminator
  alpha : Outport
  beta : Outport  Port=2
  Mach : Outport  Port=3
  q : Outport  Port=4
  wires:
  x/1 -> Bus Selector/1
  env/1 -> Bus Selector1/1
  Dynamic Pressure/1 -> q/1
  Bus Selector/1 -> Sum/1  "<Vb>"
  Mach Number/1 -> Mach/1  "Mach"
  Bus Selector1/2 -> Mach Number/2  "<a>"
  Bus Selector1/3 -> Dynamic Pressure/2  "<rho>"
  Sum/1 -> Mach Number/1, Dynamic Pressure/1, "Incidence, Sideslip, & Airspeed"/1
  "Incidence, Sideslip, & Airspeed"/1 -> alpha/1
  "Incidence, Sideslip, & Airspeed"/2 -> beta/1
  "Incidence, Sideslip, & Airspeed"/3 -> Terminator/1
  Gain/1 -> Sum/2
  Bus Selector1/1 -> Gain/1  "<ug>"

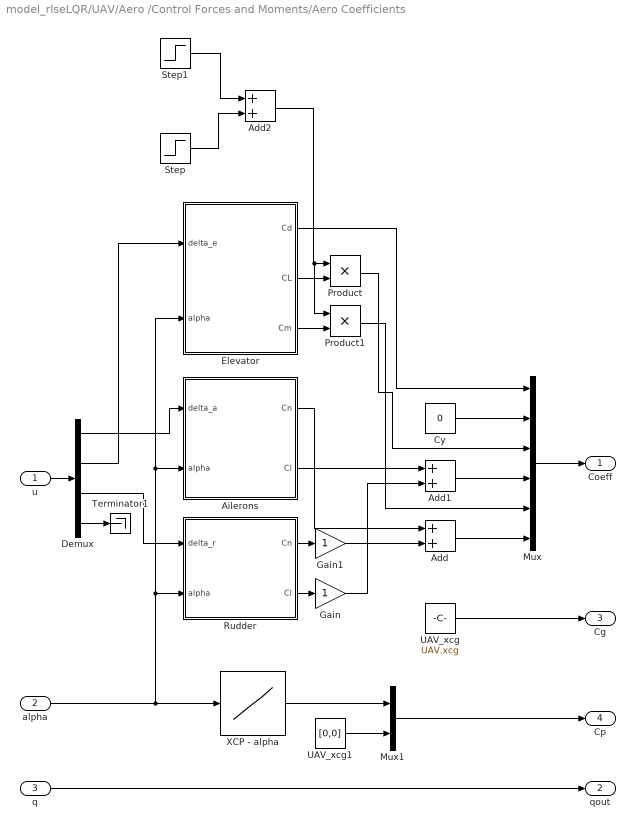
== system model_rlseLQR/UAV/Aero /Control Forces and Moments/Aero Coefficients ==
  u : Inport
  alpha : Inport  Port=2
  q : Inport  Port=3
  Add : Sum
  Add1 : Sum
  Add2 : Sum
  Ailerons : Subsystem
  Cy : Constant  Value=0
  Demux : Demux
  Elevator : Subsystem
  Gain : Gain
  Gain1 : Gain
  Mux : Mux  Inputs=6
  Mux1 : Mux  Inputs=2
  Product : Product
  Product1 : Product
  Rudder : Subsystem
  Step : Step  Time=10  Before=2  After=2  SampleTime=0
  Step1 : Step  Time=10  After=0  SampleTime=0
  Terminator1 : Terminator
  UAV_xcg : Constant  Value=UAV.xcg
  UAV_xcg1 : Constant  Value=[0,0]
  XCP - alpha : Lookup_n-D  NumberOfTableDimensions=1  BreakpointsForDimension1=UAV.alpha  Table=UAV.xcp  InternalRulePriority=Speed  RndMeth=Simplest  InputSameDT=on
  "Coeff " : Outport
  qout : Outport  Port=2
  "Cg " : Outport  Port=3
  "Cp " : Outport  Port=4
  wires:
  q/1 -> qout/1
  alpha/1 -> Rudder/2(alpha), Elevator/2(alpha), Ailerons/2(alpha), XCP - alpha/1
  u/1 -> Demux/1
  Elevator/3(Cm) -> Product1/2
  Elevator/2(CL) -> Product/2
  Demux/1 -> Ailerons/1(delta_a)
  Elevator/1(Cd) -> Mux/1
  Demux/4 -> Terminator1/1
  Cy/1 -> Mux/2
  Demux/3 -> Rudder/1(delta_r)
  Add/1 -> Mux/6
  Ailerons/1(Cn) -> Add/1
  Rudder/1(Cn) -> Gain1/1
  Add1/1 -> Mux/4
  Ailerons/2(Cl) -> Add1/1
  Rudder/2(Cl) -> Gain/1
  UAV_xcg/1 -> "Cg "/1
  Mux1/1 -> "Cp "/1
  XCP - alpha/1 -> Mux1/1
  UAV_xcg1/1 -> Mux1/2
  Mux/1 -> "Coeff "/1
  Demux/2 -> Elevator/1(delta_e)
  Gain/1 -> Add1/2
  Gain1/1 -> Add/2
  Product/1 -> Mux/3
  Product1/1 -> Mux/5
  Step/1 -> Add2/2
  Add2/1 -> Product1/1, Product/1
  Step1/1 -> Add2/1

== system model_rlseLQR/UAV/Aero /Control Forces and Moments/Aero Coefficients/Ailerons ==
  delta_a : Inport
  alpha : Inport  Port=2
  angle(right) - Cl : Lookup_n-D  NumberOfTableDimensions=1  BreakpointsForDimension1=UAV.deltar  Table=UAV.clroll  InternalRulePriority=Speed  RndMeth=Simplest  InputSameDT=on
  angle(right) - Cn : Lookup_n-D  BreakpointsForDimension1=UAV.alpha  BreakpointsForDimension2=UAV.deltar  Table=UAV.cn_asy  InternalRulePriority=Speed  RndMeth=Simplest  InputSameDT=on
  delta_a - aileron (right) angle : Lookup_n-D  NumberOfTableDimensions=1  BreakpointsForDimension1=linspace(-1,1,UAV.ndelta)  Table=UAV.deltal  InternalRulePriority=Speed  RndMeth=Simplest  InputSameDT=on
  Cn : Outport
  Cl : Outport  Port=2
  wires:
  delta_a/1 -> delta_a - aileron (right) angle/1
  angle(right) - Cl/1 -> Cl/1
  delta_a - aileron (right) angle/1 -> angle(right) - Cn/2, angle(right) - Cl/1  "Surface angle"
  alpha/1 -> angle(right) - Cn/1
  angle(right) - Cn/1 -> Cn/1

== system model_rlseLQR/UAV/Aero /Control Forces and Moments/Aero Coefficients/Elevator ==
  delta_e : Inport
  alpha : Inport  Port=2
  Product : Product
  Product1 : Product
  Product2 : Product
  alpha - q/qinf : Lookup_n-D  NumberOfTableDimensions=1  BreakpointsForDimension1=UAV.alpha  Table=UAV.qqinf  InternalRulePriority=Speed  RndMeth=Simplest  InputSameDT=on
  dc_delta_e : Lookup_n-D  BreakpointsForDimension1=UAV.alpha  BreakpointsForDimension2=UAV.delta  Table=UAV.dcdi_sym  InternalRulePriority=Speed  RndMeth=Simplest  InputSameDT=on
  dcl_delta_e : Lookup_n-D  NumberOfTableDimensions=1  BreakpointsForDimension1=UAV.delta  Table=UAV.dcl_sym  InternalRulePriority=Speed  RndMeth=Simplest  InputSameDT=on
  dcm_delta_e : Lookup_n-D  NumberOfTableDimensions=1  BreakpointsForDimension1=UAV.delta  Table=UAV.dcm_sym  InternalRulePriority=Speed  RndMeth=Simplest  InputSameDT=on
  delta_e - elevator angle : Lookup_n-D  NumberOfTableDimensions=1  BreakpointsForDimension1=linspace(-1,1,UAV.ndelta)  Table=UAV.delta  InternalRulePriority=Speed  RndMeth=Simplest  InputSameDT=on
  Cd : Outport
  CL : Outport  Port=2
  Cm : Outport  Port=3
  wires:
  delta_e/1 -> delta_e - elevator angle/1
  delta_e - elevator angle/1 -> dc_delta_e/2, dcl_delta_e/1, dcm_delta_e/1  "Surface angle"
  dcm_delta_e/1 -> Product/1
  Product/1 -> Cm/1
  Product1/1 -> CL/1
  dcl_delta_e/1 -> Product1/1
  alpha - q/qinf/1 -> Product2/2, Product/2, Product1/2  "Surface angle"
  alpha/1 -> dc_delta_e/1, alpha - q/qinf/1
  Product2/1 -> Cd/1
  dc_delta_e/1 -> Product2/1

== system model_rlseLQR/UAV/Aero /Control Forces and Moments/Aero Coefficients/Rudder ==
  delta_r : Inport
  alpha : Inport  Port=2
  - h_alpha/B : Lookup_n-D  NumberOfTableDimensions=1  BreakpointsForDimension1=UAV.alpha  Table=UAV.hrudder_a  InternalRulePriority=Speed  RndMeth=Simplest  InputSameDT=on
  Multiply : Product
  Srudder/Sref : Gain  Gain=UAV.srudder_a
  deg2rad * 2pi (CL) : Gain  Gain=(2*pi)^2/360
  l_rudder/l_ref : Gain  Gain=UAV.lrudder_a
  "u_r -> deg" : Gain  Gain=UAV.delta_rud_max
  Cn : Outport
  Cl : Outport  Port=2
  wires:
  deg2rad * 2pi (CL)/1 -> Srudder/Sref/1  "CL"
  Srudder/Sref/1 -> Multiply/1, l_rudder/l_ref/1
  l_rudder/l_ref/1 -> Cn/1
  "u_r -> deg"/1 -> deg2rad * 2pi (CL)/1
  delta_r/1 -> "u_r -> deg"/1
  alpha/1 -> - h_alpha/B/1
  - h_alpha/B/1 -> Multiply/2
  Multiply/1 -> Cl/1

== matlab function model_rlseLQR/Controller/RLSE - K_long/RLSE & LQR/MATLAB Function ==
  data: A input; Aout output; B input; DX_err input; XU input; P input; Bout output; P output
function [Aout,Bout,P] = RLSE_klm_long(A,B,DX_err,XU,P)
    % Re calculate A and B matrices from the new data point
    Aout = zeros(4);
    Bout = zeros(4,2);
    R = 1;
    I = eye(6);
    
    AB = [A B];
    AB = AB';

    K = P*XU/(XU'*P*XU + R);
    P = (I-K*XU')*P;
    
    AB = AB + K*(DX_err');
    
    AB = AB';
    Aout = AB(:,1:4);
    Bout = AB(:,5:6);
end

== matlab function model_rlseLQR/Random input/random imput vector ==
  data: y output
function y = rand_u
y = (rand(4,1) -0.5*ones(4,1)).*[0.1;0.1;0.1;0.2];
